simulink model "identification_LQR_closed"  (R2019b)
settings: Solver=FixedStepAuto  StartTime=0.0  StopTime=inf  FixedStep=0.01  RelTol=1e-3
values from neighbouring files (symbols this model uses):
  Kw = 1/(sys_dis.C*inv(eye(2) - sys_dis.A + sys_dis.B*K)*sys_dis.B)    [controller_LQR_tryout.m]
undefined symbols (not defined in the file or in its folder): K
libraries: simulink x1, sldrtlib x1
settings Model: Creator=mandl  LastModifiedBy=mandl
settings SolverCC: AlgebraicLoopSolver=LineSearch

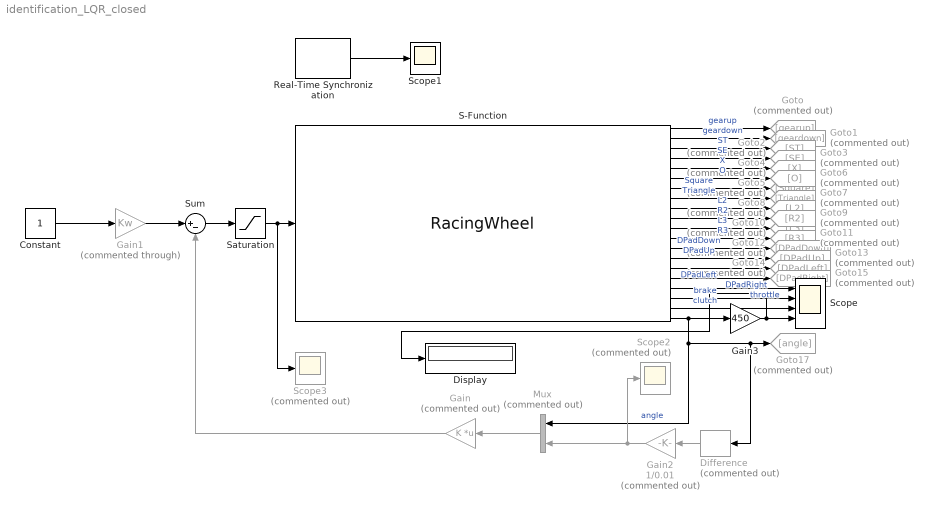
== system identification_LQR_closed ==
  Constant : Constant
  Difference : simulink/Discrete/Difference  Commented=on  ICPrevInput=0.0  OutMin=[]  OutMax=[]  OutDataType=fixdt(1, 16)  OutScaling=2^-10  DoSatur=off
  Display : Display
  Gain : Gain  Commented=on  Gain=K  Multiplication=Matrix(K*u)
  Gain1 : Gain  Commented=through  Gain=Kw
  Gain2 : Gain  Commented=on  Gain=1/0.01
  Gain3 : Gain  Gain=450
  Goto : Goto  Commented=on  GotoTag=gearup
  Goto1 : Goto  Commented=on  GotoTag=geardown
  Goto10 : Goto  Commented=on  GotoTag=L3
  Goto11 : Goto  Commented=on  GotoTag=R3
  Goto12 : Goto  Commented=on  GotoTag=DPadDown
  Goto13 : Goto  Commented=on  GotoTag=DPadUp
  Goto14 : Goto  Commented=on  GotoTag=DPadLeft
  Goto15 : Goto  Commented=on  GotoTag=DPadRight
  Goto17 : Goto  Commented=on  GotoTag=angle
  Goto2 : Goto  Commented=on  GotoTag=ST
  Goto3 : Goto  Commented=on  GotoTag=SE
  Goto4 : Goto  Commented=on  GotoTag=X
  Goto5 : Goto  Commented=on  GotoTag=Square
  Goto6 : Goto  Commented=on  GotoTag=O
  Goto7 : Goto  Commented=on  GotoTag=Triangle
  Goto8 : Goto  Commented=on  GotoTag=L2
  Goto9 : Goto  Commented=on  GotoTag=R2
  Mux : Mux  Commented=on  Inputs=2
  Real-Time Synchronization : sldrtlib/Real-Time Synchronization  SampleTime=0.01  MaxMissedTicks=100  ShowMissedTicks=on  YieldWhenWaiting=off
  S-Function : S-Function  FunctionName=RacingWheel  Parameters=Ts_FF  SFunctionModules=RacingWheel_wrapper  SFunctionDeploymentMode=off  EnableBusSupport=off  mask(Racing Wheel with Force Feedback){Ts_FF=0.01}
      mask prompts: Ts_FF "Constant Force-Feedback Sample Time"
      mask help: Interacts with the windows gaming API from UWP. The force feedback effect is constant over the user defined sampling time below.
      mask init:
      | val = [[.9  0.75 0.75 1 1 .9 .9 1]',[1 1 0.75 0.75 .9 .9 1 .9]'];try , sys = get_param(gcb,'SfunBuilderFcnName');if isempty(sys), sys = get_param(gcb,'FunctionName'); end,catch, sys = get_param(gcb,'FunctionName'); end
      mask Display:
      | plot(val(:,1),val(:,2)),disp(sys),
      | image('icon.png'),
      | port_label('input',1,'FF'),
      | port_label('output',1,'gearup'),
      | port_label('output',2,'geardown'),
      | port_label('output',3,'ST'),
      | port_label('output',4,'SE'),
      | port_label('output',5,'X'),
      | port_label('output',6,'O'),
      | port_label('output',7,'Square'),
      | port_label('output',8,'Triangle'),
      | port_label('output',9,'L2'),
      | port_label('output',10,'R2'),
      | port_label('output',11,'L3'),
      | port_label('output',12,'R3'),
      | port_label('output',13,'DPadDown'),
      | port_label('output',14,'DPadUp'),
      | port_label('output',15,'DPadLeft'),
      | port_label('output',16,'DPadRight'),
      | port_label('output',17,'throttle'),
      | port_label('output',18,'brake'),
      | port_label('output',19,'clutch'),
      | port_label('output',20,'angle')
  Saturation : Saturate  UpperLimit=1  LowerLimit=-1
  Scope : Scope  NumInputPorts=4
  Scope1 : Scope
  Scope2 : Scope  Commented=on
  Scope3 : Scope  Commented=on
  Sum : Sum  Inputs=|+-
  wires:
  S-Function/20 -> Difference/1, Goto17/1, Mux/1, Gain3/1  "angle"
  S-Function/19 -> Scope/3  "clutch"
  S-Function/18 -> Scope/2  "brake"
  S-Function/17 -> Scope/1  "throttle"
  S-Function/1 -> Goto/1  "gearup"
  S-Function/2 -> Goto1/1  "geardown"
  S-Function/3 -> Goto2/1  "ST"
  S-Function/4 -> Goto3/1  "SE"
  S-Function/5 -> Goto4/1  "X"
  S-Function/6 -> Goto6/1  "O"
  S-Function/7 -> Goto5/1  "Square"
  S-Function/8 -> Goto7/1  "Triangle"
  S-Function/9 -> Goto8/1  "L2"
  S-Function/10 -> Goto9/1  "R2"
  S-Function/11 -> Goto10/1  "L3"
  S-Function/12 -> Goto11/1  "R3"
  S-Function/13 -> Goto12/1  "DPadDown"
  S-Function/14 -> Goto13/1  "DPadUp"
  S-Function/15 -> Goto14/1  "DPadLeft"
  S-Function/16 -> Goto15/1  "DPadRight"
  Real-Time Synchronization/1 -> Scope1/1
  Constant/1 -> Gain1/1
  Gain1/1 -> Sum/1
  Gain/1 -> Sum/2
  Mux/1 -> Gain/1
  Difference/1 -> Gain2/1
  Sum/1 -> Saturation/1
  Saturation/1 -> Scope3/1, S-Function/1
  Gain2/1 -> Scope2/1, Mux/2
  Gain3/1 -> Display/1, Scope/4
